simulink model "s2_0515"  (R2016a)
settings: Solver=ode23tb  StartTime=0.0  StopTime=40e-6  MaxStep=0.2  RelTol=1e-4
PreLoadFcn:
  | % -- Recommended Settings --
  | %
  | %  Simulink:
  | %      Solver: Ode23tb
  | %      Relative tolerance = 1e-4
  | %      Max step size = 0.2
  | %
  | %  Powergui:
  |          Ts = 0; % (continuous electrical model)
  | %
  | %
  | % ----------------------------------
libraries: powerlib x14
settings Model: Creator=Administrator  LastModifiedBy=Administrator
settings DataIOCC: LimitDataPoints=on
settings DebuggingCC: AllowSymbolicDim=off
settings ConfigComp: CovModelRefEnable=Off  CovSFcnEnable=off

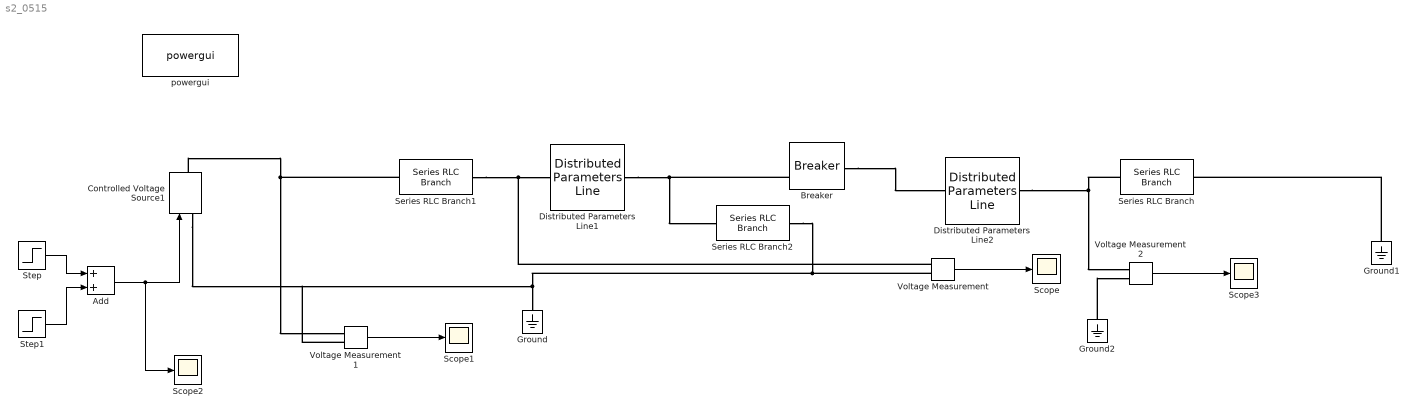
== system s2_0515 ==
  Add : Sum
  Breaker : powerlib/Elements/Breaker  InitialState=1  SwitchingTimes="[1/60  5/60]"  External=on  BreakerResistance=0.01  SnubberResistance=1e6  SnubberCapacitance=inf  Measurements=None  MoreParameters=on  NoBreakLoop=off
  Controlled Voltage Source1 : powerlib/Electrical Sources/Controlled Voltage Source  Initialize=off  Source_Type=DC  Amplitude=0  Phase=0  Frequency=0  Measurements=Voltage
  Distributed Parameters Line1 : powerlib/Elements/Distributed Parameters Line  Phases=1  Frequency=1000  Resistance=1.8E-1  Inductance=2.75E-4  Capacitance=5.57E-7  Length=0.2  x1=[-2.48e-06 0;-2.47e-06 0;-2.46e-06 0;-2.45e-06 0;-2.44e-06 0;-2.43e-06 0;-2.42e-06 0;-2.41e-06 0;-2.4e-06 0;-2.39e-06 0;-2.38e-06 0;-2.37e-06 0;-2.36e-06 0;-2.35e-06 0;-2.34e-06 0;-2.33e-06 0;-2.32e-06 0;-2.31e-06 0;-2.3e-06 0;-2.29e-06 0;-2.28e-06 0;-2.27e-06 0;-2.26e-06 0;-2.25e-06 0;-2.24e-06 0;-2.23e-06 0;-2.22e-06 0;-2.21e-06 0;-2.2e-06 0;-2.19e-06 0;-2.18e-06 0;-2.17e-06 0;-2.16e-06 0;-2.15e-06 0;-2.14e-06 0;-2.13e-06 0;-2.12e-06 0;-2.11e-06 0;-2.1e-06 0;-2.09e-06 0;-2.08e-06 0;-2.07e-06 0;-2.06e-06 0;-2.05e-06 0;-2.04e-06 0;-2.03e-06 0;-2.02e-06 0;-2.01e-06 0;-2e-06 0;-1.99e-06 0;-1.98e-06 0;-1.97e-06 0;-1.96e-06 0;-1.95e-06 0;-1.94e-06 0;-1.93e-06 0;-1.92e-06 0;-1.91e-06 0;-1.9e-06 0;-1.89e-06 0;-1.88e-06 0;-1.87e-06 0;-1.86e-06 0;-1.85e-06 0;-1.84e-06 0;-1.83e-06 0;-1.82e-06 0;-1.81e-06 0;-1.8e-06 0;-1.79e-06 0;-1.78e-06 0;-1.77e-06 0;-1.76e-06 0;-1.75e-06 0;-1.74e-06 0;-1.73e-06 0;-1.72e-06 0;-1.71e-06 0;-1.7e-06 0;-1.69e-06 0;-1.68e-06 0;-1.67e-06 0;-1.66e-06 0;-1.65e-06 0;-1.64e-06 0;-1.63e-06 0;-1.62e-06 0;-1.61e-06 0;-1.6e-06 0;-1.59e-06 0;-1.58e-06 0;-1.57e-06 0;-1.56e-06 0;-1.55e-06 0;-1.54e-06 0;-1.53e-06 0;-1.52e-06 0;-1.51e-06 0;-1.5e-06 0;-1.49e-06 0;-1.48e-06 0;-1.47e-06 0;-1.46e-06 0;-1.45e-06 0;-1.44e-06 0;-1.43e-06 0;-1.42e-06 0;-1.41e-06 0;-1.4e-06 0;-1.39e-06 0;-1.38e-06 0;-1.37e-06 0;-1.36e-06 0;-1.35e-06 0;-1.34e-06 0;-1.33e-06 0;-1.32e-06 0;-1.31e-06 0;-1.3e-06 0;-1.29e-06 0;-1.28e-06 0;-1.27e-06 0;-1.26e-06 0;-1.25e-06 0;-1.24e-06 0;-1.23e-06 0;-1.22e-06 0;-1.21e-06 0;-1.2e-06 0;-1.19e-06 0;-1.18e-06 0;-1.17e-06 0;-1.16e-06 0;-1.15e-06 0;-1.14e-06 0;-1.13e-06 0;-1.12e-06 0;-1.11e-06 0;-1.1e-06 0;-1.09e-06 0;-1.08e-06 0;-1.07e-06 0;-1.06e-06 0;-1.05e-06 0;-1.04e-06 0;-1.03e-06 0;-1.02e-06 0;-1.01e-06 0;-1e-06 0;-9.9e-07 0;-9.8e-07 0;-9.7e-07 0;-9.6e-07 0;-9.5e-07 0;-9.4e-07 0;-9.3e-07 0;-9.2e-07 0;-9.1e-07 0;-9e-07 0;-8.9e-07 0;-8.8e-07 0;-8.7e-07 0;-8.6e-07 0;-8.5e-07 0;-8.4e-07 0;-8.3e-07 0;-8.2e-07 0;-8.1e-07 0;-8e-07 0;-7.9e-07 0;-7.8e-07 0;-7.7e-07 0;-7.6e-07 0;-7.5e-07 0;-7.4e-07 0;-7.3e-07 0;-7.2e-07 0;-7.1e-07 0;-7e-07 0;-6.9e-07 0;-6.8e-07 0;-6.7e-07 0;-6.6e-07 0;-6.5e-07 0;-6.4e-07 0;-6.3e-07 0;-6.2e-07 0;-6.1e-07 0;-6e-07 0;-5.9e-07 0;-5.8e-07 0;-5.7e-07 0;-5.6e-07 0;-5.5e-07 0;-5.4e-07 0;-5.3e-07 0;-5.2e-07 0;-5.1e-07 0;-5e-07 0;-4.9e-07 0;-4.8e-07 0;-4.7e-07 0;-4.6e-07 0;-4.5e-07 0;-4.4e-07 0;-4.3e-07 0;-4.2e-07 0;-4.1e-07 0;-4e-07 0;-3.9e-07 0;-3.8e-07 0;-3.7e-07 0;-3.6e-07 0;-3.5e-07 0;-3.4e-07 0;-3.3e-07 0;-3.2e-07 0;-3.1e-07 0;-3e-07 0;-2.9e-07 0;-2.8e-07 0;-2.7e-07 0;-2.6e-07 0;-2.5e-07 0;-2.4e-07 0;-2.3e-07 0;-2.2e-07 0;-2.1e-07 0;-2e-07 0;-1.9e-07 0;-1.8e-07 0;-1.7e-07 0;-1.6e-07 0;-1.5e-07 0;-1.4e-07 0;-1.3e-07 0;-1.2e-07 0;-1.1e-07 0;-1e-07 0;-9e-08 0;-8e-08 0;-7e-08 0;-6e-08 0;-5e-08 0;-4e-08 0;-3e-08 0;-2e-08 0;-1e-08 0]  x2=[-2.48e-06 0;-2.47e-06 0;-2.46e-06 0;-2.45e-06 0;-2.44e-06 0;-2.43e-06 0;-2.42e-06 0;-2.41e-06 0;-2.4e-06 0;-2.39e-06 0;-2.38e-06 0;-2.37e-06 0;-2.36e-06 0;-2.35e-06 0;-2.34e-06 0;-2.33e-06 0;-2.32e-06 0;-2.31e-06 0;-2.3e-06 0;-2.29e-06 0;-2.28e-06 0;-2.27e-06 0;-2.26e-06 0;-2.25e-06 0;-2.24e-06 0;-2.23e-06 0;-2.22e-06 0;-2.21e-06 0;-2.2e-06 0;-2.19e-06 0;-2.18e-06 0;-2.17e-06 0;-2.16e-06 0;-2.15e-06 0;-2.14e-06 0;-2.13e-06 0;-2.12e-06 0;-2.11e-06 0;-2.1e-06 0;-2.09e-06 0;-2.08e-06 0;-2.07e-06 0;-2.06e-06 0;-2.05e-06 0;-2.04e-06 0;-2.03e-06 0;-2.02e-06 0;-2.01e-06 0;-2e-06 0;-1.99e-06 0;-1.98e-06 0;-1.97e-06 0;-1.96e-06 0;-1.95e-06 0;-1.94e-06 0;-1.93e-06 0;-1.92e-06 0;-1.91e-06 0;-1.9e-06 0;-1.89e-06 0;-1.88e-06 0;-1.87e-06 0;-1.86e-06 0;-1.85e-06 0;-1.84e-06 0;-1.83e-06 0;-1.82e-06 0;-1.81e-06 0;-1.8e-06 0;-1.79e-06 0;-1.78e-06 0;-1.77e-06 0;-1.76e-06 0;-1.75e-06 0;-1.74e-06 0;-1.73e-06 0;-1.72e-06 0;-1.71e-06 0;-1.7e-06 0;-1.69e-06 0;-1.68e-06 0;-1.67e-06 0;-1.66e-06 0;-1.65e-06 0;-1.64e-06 0;-1.63e-06 0;-1.62e-06 0;-1.61e-06 0;-1.6e-06 0;-1.59e-06 0;-1.58e-06 0;-1.57e-06 0;-1.56e-06 0;-1.55e-06 0;-1.54e-06 0;-1.53e-06 0;-1.52e-06 0;-1.51e-06 0;-1.5e-06 0;-1.49e-06 0;-1.48e-06 0;-1.47e-06 0;-1.46e-06 0;-1.45e-06 0;-1.44e-06 0;-1.43e-06 0;-1.42e-06 0;-1.41e-06 0;-1.4e-06 0;-1.39e-06 0;-1.38e-06 0;-1.37e-06 0;-1.36e-06 0;-1.35e-06 0;-1.34e-06 0;-1.33e-06 0;-1.32e-06 0;-1.31e-06 0;-1.3e-06 0;-1.29e-06 0;-1.28e-06 0;-1.27e-06 0;-1.26e-06 0;-1.25e-06 0;-1.24e-06 0;-1.23e-06 0;-1.22e-06 0;-1.21e-06 0;-1.2e-06 0;-1.19e-06 0;-1.18e-06 0;-1.17e-06 0;-1.16e-06 0;-1.15e-06 0;-1.14e-06 0;-1.13e-06 0;-1.12e-06 0;-1.11e-06 0;-1.1e-06 0;-1.09e-06 0;-1.08e-06 0;-1.07e-06 0;-1.06e-06 0;-1.05e-06 0;-1.04e-06 0;-1.03e-06 0;-1.02e-06 0;-1.01e-06 0;-1e-06 0;-9.9e-07 0;-9.8e-07 0;-9.7e-07 0;-9.6e-07 0;-9.5e-07 0;-9.4e-07 0;-9.3e-07 0;-9.2e-07 0;-9.1e-07 0;-9e-07 0;-8.9e-07 0;-8.8e-07 0;-8.7e-07 0;-8.6e-07 0;-8.5e-07 0;-8.4e-07 0;-8.3e-07 0;-8.2e-07 0;-8.1e-07 0;-8e-07 0;-7.9e-07 0;-7.8e-07 0;-7.7e-07 0;-7.6e-07 0;-7.5e-07 0;-7.4e-07 0;-7.3e-07 0;-7.2e-07 0;-7.1e-07 0;-7e-07 0;-6.9e-07 0;-6.8e-07 0;-6.7e-07 0;-6.6e-07 0;-6.5e-07 0;-6.4e-07 0;-6.3e-07 0;-6.2e-07 0;-6.1e-07 0;-6e-07 0;-5.9e-07 0;-5.8e-07 0;-5.7e-07 0;-5.6e-07 0;-5.5e-07 0;-5.4e-07 0;-5.3e-07 0;-5.2e-07 0;-5.1e-07 0;-5e-07 0;-4.9e-07 0;-4.8e-07 0;-4.7e-07 0;-4.6e-07 0;-4.5e-07 0;-4.4e-07 0;-4.3e-07 0;-4.2e-07 0;-4.1e-07 0;-4e-07 0;-3.9e-07 0;-3.8e-07 0;-3.7e-07 0;-3.6e-07 0;-3.5e-07 0;-3.4e-07 0;-3.3e-07 0;-3.2e-07 0;-3.1e-07 0;-3e-07 0;-2.9e-07 0;-2.8e-07 0;-2.7e-07 0;-2.6e-07 0;-2.5e-07 0;-2.4e-07 0;-2.3e-07 0;-2.2e-07 0;-2.1e-07 0;-2e-07 0;-1.9e-07 0;-1.8e-07 0;-1.7e-07 0;-1.6e-07 0;-1.5e-07 0;-1.4e-07 0;-1.3e-07 0;-1.2e-07 0;-1.1e-07 0;-1e-07 0;-9e-08 0;-8e-08 0;-7e-08 0;-6e-08 0;-5e-08 0;-4e-08 0;-3e-08 0;-2e-08 0;-1e-08 0]  x3=[-2.48e-06 0;-2.47e-06 0;-2.46e-06 0;-2.45e-06 0;-2.44e-06 0;-2.43e-06 0;-2.42e-06 0;-2.41e-06 0;-2.4e-06 0;-2.39e-06 0;-2.38e-06 0;-2.37e-06 0;-2.36e-06 0;-2.35e-06 0;-2.34e-06 0;-2.33e-06 0;-2.32e-06 0;-2.31e-06 0;-2.3e-06 0;-2.29e-06 0;-2.28e-06 0;-2.27e-06 0;-2.26e-06 0;-2.25e-06 0;-2.24e-06 0;-2.23e-06 0;-2.22e-06 0;-2.21e-06 0;-2.2e-06 0;-2.19e-06 0;-2.18e-06 0;-2.17e-06 0;-2.16e-06 0;-2.15e-06 0;-2.14e-06 0;-2.13e-06 0;-2.12e-06 0;-2.11e-06 0;-2.1e-06 0;-2.09e-06 0;-2.08e-06 0;-2.07e-06 0;-2.06e-06 0;-2.05e-06 0;-2.04e-06 0;-2.03e-06 0;-2.02e-06 0;-2.01e-06 0;-2e-06 0;-1.99e-06 0;-1.98e-06 0;-1.97e-06 0;-1.96e-06 0;-1.95e-06 0;-1.94e-06 0;-1.93e-06 0;-1.92e-06 0;-1.91e-06 0;-1.9e-06 0;-1.89e-06 0;-1.88e-06 0;-1.87e-06 0;-1.86e-06 0;-1.85e-06 0;-1.84e-06 0;-1.83e-06 0;-1.82e-06 0;-1.81e-06 0;-1.8e-06 0;-1.79e-06 0;-1.78e-06 0;-1.77e-06 0;-1.76e-06 0;-1.75e-06 0;-1.74e-06 0;-1.73e-06 0;-1.72e-06 0;-1.71e-06 0;-1.7e-06 0;-1.69e-06 0;-1.68e-06 0;-1.67e-06 0;-1.66e-06 0;-1.65e-06 0;-1.64e-06 0;-1.63e-06 0;-1.62e-06 0;-1.61e-06 0;-1.6e-06 0;-1.59e-06 0;-1.58e-06 0;-1.57e-06 0;-1.56e-06 0;-1.55e-06 0;-1.54e-06 0;-1.53e-06 0;-1.52e-06 0;-1.51e-06 0;-1.5e-06 0;-1.49e-06 0;-1.48e-06 0;-1.47e-06 0;-1.46e-06 0;-1.45e-06 0;-1.44e-06 0;-1.43e-06 0;-1.42e-06 0;-1.41e-06 0;-1.4e-06 0;-1.39e-06 0;-1.38e-06 0;-1.37e-06 0;-1.36e-06 0;-1.35e-06 0;-1.34e-06 0;-1.33e-06 0;-1.32e-06 0;-1.31e-06 0;-1.3e-06 0;-1.29e-06 0;-1.28e-06 0;-1.27e-06 0;-1.26e-06 0;-1.25e-06 0;-1.24e-06 0;-1.23e-06 0;-1.22e-06 0;-1.21e-06 0;-1.2e-06 0;-1.19e-06 0;-1.18e-06 0;-1.17e-06 0;-1.16e-06 0;-1.15e-06 0;-1.14e-06 0;-1.13e-06 0;-1.12e-06 0;-1.11e-06 0;-1.1e-06 0;-1.09e-06 0;-1.08e-06 0;-1.07e-06 0;-1.06e-06 0;-1.05e-06 0;-1.04e-06 0;-1.03e-06 0;-1.02e-06 0;-1.01e-06 0;-1e-06 0;-9.9e-07 0;-9.8e-07 0;-9.7e-07 0;-9.6e-07 0;-9.5e-07 0;-9.4e-07 0;-9.3e-07 0;-9.2e-07 0;-9.1e-07 0;-9e-07 0;-8.9e-07 0;-8.8e-07 0;-8.7e-07 0;-8.6e-07 0;-8.5e-07 0;-8.4e-07 0;-8.3e-07 0;-8.2e-07 0;-8.1e-07 0;-8e-07 0;-7.9e-07 0;-7.8e-07 0;-7.7e-07 0;-7.6e-07 0;-7.5e-07 0;-7.4e-07 0;-7.3e-07 0;-7.2e-07 0;-7.1e-07 0;-7e-07 0;-6.9e-07 0;-6.8e-07 0;-6.7e-07 0;-6.6e-07 0;-6.5e-07 0;-6.4e-07 0;-6.3e-07 0;-6.2e-07 0;-6.1e-07 0;-6e-07 0;-5.9e-07 0;-5.8e-07 0;-5.7e-07 0;-5.6e-07 0;-5.5e-07 0;-5.4e-07 0;-5.3e-07 0;-5.2e-07 0;-5.1e-07 0;-5e-07 0;-4.9e-07 0;-4.8e-07 0;-4.7e-07 0;-4.6e-07 0;-4.5e-07 0;-4.4e-07 0;-4.3e-07 0;-4.2e-07 0;-4.1e-07 0;-4e-07 0;-3.9e-07 0;-3.8e-07 0;-3.7e-07 0;-3.6e-07 0;-3.5e-07 0;-3.4e-07 0;-3.3e-07 0;-3.2e-07 0;-3.1e-07 0;-3e-07 0;-2.9e-07 0;-2.8e-07 0;-2.7e-07 0;-2.6e-07 0;-2.5e-07 0;-2.4e-07 0;-2.3e-07 0;-2.2e-07 0;-2.1e-07 0;-2e-07 0;-1.9e-07 0;-1.8e-07 0;-1.7e-07 0;-1.6e-07 0;-1.5e-07 0;-1.4e-07 0;-1.3e-07 0;-1.2e-07 0;-1.1e-07 0;-1e-07 0;-9e-08 0;-8e-08 0;-7e-08 0;-6e-08 0;-5e-08 0;-4e-08 0;-3e-08 0;-2e-08 0;-1e-08 0]  x4=[-2.48e-06 0;-2.47e-06 0;-2.46e-06 0;-2.45e-06 0;-2.44e-06 0;-2.43e-06 0;-2.42e-06 0;-2.41e-06 0;-2.4e-06 0;-2.39e-06 0;-2.38e-06 0;-2.37e-06 0;-2.36e-06 0;-2.35e-06 0;-2.34e-06 0;-2.33e-06 0;-2.32e-06 0;-2.31e-06 0;-2.3e-06 0;-2.29e-06 0;-2.28e-06 0;-2.27e-06 0;-2.26e-06 0;-2.25e-06 0;-2.24e-06 0;-2.23e-06 0;-2.22e-06 0;-2.21e-06 0;-2.2e-06 0;-2.19e-06 0;-2.18e-06 0;-2.17e-06 0;-2.16e-06 0;-2.15e-06 0;-2.14e-06 0;-2.13e-06 0;-2.12e-06 0;-2.11e-06 0;-2.1e-06 0;-2.09e-06 0;-2.08e-06 0;-2.07e-06 0;-2.06e-06 0;-2.05e-06 0;-2.04e-06 0;-2.03e-06 0;-2.02e-06 0;-2.01e-06 0;-2e-06 0;-1.99e-06 0;-1.98e-06 0;-1.97e-06 0;-1.96e-06 0;-1.95e-06 0;-1.94e-06 0;-1.93e-06 0;-1.92e-06 0;-1.91e-06 0;-1.9e-06 0;-1.89e-06 0;-1.88e-06 0;-1.87e-06 0;-1.86e-06 0;-1.85e-06 0;-1.84e-06 0;-1.83e-06 0;-1.82e-06 0;-1.81e-06 0;-1.8e-06 0;-1.79e-06 0;-1.78e-06 0;-1.77e-06 0;-1.76e-06 0;-1.75e-06 0;-1.74e-06 0;-1.73e-06 0;-1.72e-06 0;-1.71e-06 0;-1.7e-06 0;-1.69e-06 0;-1.68e-06 0;-1.67e-06 0;-1.66e-06 0;-1.65e-06 0;-1.64e-06 0;-1.63e-06 0;-1.62e-06 0;-1.61e-06 0;-1.6e-06 0;-1.59e-06 0;-1.58e-06 0;-1.57e-06 0;-1.56e-06 0;-1.55e-06 0;-1.54e-06 0;-1.53e-06 0;-1.52e-06 0;-1.51e-06 0;-1.5e-06 0;-1.49e-06 0;-1.48e-06 0;-1.47e-06 0;-1.46e-06 0;-1.45e-06 0;-1.44e-06 0;-1.43e-06 0;-1.42e-06 0;-1.41e-06 0;-1.4e-06 0;-1.39e-06 0;-1.38e-06 0;-1.37e-06 0;-1.36e-06 0;-1.35e-06 0;-1.34e-06 0;-1.33e-06 0;-1.32e-06 0;-1.31e-06 0;-1.3e-06 0;-1.29e-06 0;-1.28e-06 0;-1.27e-06 0;-1.26e-06 0;-1.25e-06 0;-1.24e-06 0;-1.23e-06 0;-1.22e-06 0;-1.21e-06 0;-1.2e-06 0;-1.19e-06 0;-1.18e-06 0;-1.17e-06 0;-1.16e-06 0;-1.15e-06 0;-1.14e-06 0;-1.13e-06 0;-1.12e-06 0;-1.11e-06 0;-1.1e-06 0;-1.09e-06 0;-1.08e-06 0;-1.07e-06 0;-1.06e-06 0;-1.05e-06 0;-1.04e-06 0;-1.03e-06 0;-1.02e-06 0;-1.01e-06 0;-1e-06 0;-9.9e-07 0;-9.8e-07 0;-9.7e-07 0;-9.6e-07 0;-9.5e-07 0;-9.4e-07 0;-9.3e-07 0;-9.2e-07 0;-9.1e-07 0;-9e-07 0;-8.9e-07 0;-8.8e-07 0;-8.7e-07 0;-8.6e-07 0;-8.5e-07 0;-8.4e-07 0;-8.3e-07 0;-8.2e-07 0;-8.1e-07 0;-8e-07 0;-7.9e-07 0;-7.8e-07 0;-7.7e-07 0;-7.6e-07 0;-7.5e-07 0;-7.4e-07 0;-7.3e-07 0;-7.2e-07 0;-7.1e-07 0;-7e-07 0;-6.9e-07 0;-6.8e-07 0;-6.7e-07 0;-6.6e-07 0;-6.5e-07 0;-6.4e-07 0;-6.3e-07 0;-6.2e-07 0;-6.1e-07 0;-6e-07 0;-5.9e-07 0;-5.8e-07 0;-5.7e-07 0;-5.6e-07 0;-5.5e-07 0;-5.4e-07 0;-5.3e-07 0;-5.2e-07 0;-5.1e-07 0;-5e-07 0;-4.9e-07 0;-4.8e-07 0;-4.7e-07 0;-4.6e-07 0;-4.5e-07 0;-4.4e-07 0;-4.3e-07 0;-4.2e-07 0;-4.1e-07 0;-4e-07 0;-3.9e-07 0;-3.8e-07 0;-3.7e-07 0;-3.6e-07 0;-3.5e-07 0;-3.4e-07 0;-3.3e-07 0;-3.2e-07 0;-3.1e-07 0;-3e-07 0;-2.9e-07 0;-2.8e-07 0;-2.7e-07 0;-2.6e-07 0;-2.5e-07 0;-2.4e-07 0;-2.3e-07 0;-2.2e-07 0;-2.1e-07 0;-2e-07 0;-1.9e-07 0;-1.8e-07 0;-1.7e-07 0;-1.6e-07 0;-1.5e-07 0;-1.4e-07 0;-1.3e-07 0;-1.2e-07 0;-1.1e-07 0;-1e-07 0;-9e-08 0;-8e-08 0;-7e-08 0;-6e-08 0;-5e-08 0;-4e-08 0;-3e-08 0;-2e-08 0;-1e-08 0]  x5=2.47527776219155e-06  V1=[0;0;1.571]  V2=[0;0;1.571]  I1=[0;0;1.571]  I2=[0;0;1.571]  nHarmo=1  Measurements=Phase-to-ground voltages
  Distributed Parameters Line2 : powerlib/Elements/Distributed Parameters Line  Phases=1  Frequency=1000  Resistance=1.8E-1  Inductance=2.75E-4  Capacitance=5.57E-7  Length=0.8  x1=[-9.91e-06 0;-9.9e-06 0;-9.89e-06 0;-9.88e-06 0;-9.87e-06 0;-9.86e-06 0;-9.85e-06 0;-9.84e-06 0;-9.83e-06 0;-9.82e-06 0;-9.81e-06 0;-9.8e-06 0;-9.79e-06 0;-9.78e-06 0;-9.77e-06 0;-9.76e-06 0;-9.75e-06 0;-9.74e-06 0;-9.73e-06 0;-9.72e-06 0;-9.71e-06 0;-9.7e-06 0;-9.69e-06 0;-9.68e-06 0;-9.67e-06 0;-9.66e-06 0;-9.65e-06 0;-9.64e-06 0;-9.63e-06 0;-9.62e-06 0;-9.61e-06 0;-9.6e-06 0;-9.59e-06 0;-9.58e-06 0;-9.57e-06 0;-9.56e-06 0;-9.55e-06 0;-9.54e-06 0;-9.53e-06 0;-9.52e-06 0;-9.51e-06 0;-9.5e-06 0;-9.49e-06 0;-9.48e-06 0;-9.47e-06 0;-9.46e-06 0;-9.45e-06 0;-9.44e-06 0;-9.43e-06 0;-9.42e-06 0;-9.41e-06 0;-9.4e-06 0;-9.39e-06 0;-9.38e-06 0;-9.37e-06 0;-9.36e-06 0;-9.35e-06 0;-9.34e-06 0;-9.33e-06 0;-9.32e-06 0;-9.31e-06 0;-9.3e-06 0;-9.29e-06 0;-9.28e-06 0;-9.27e-06 0;-9.26e-06 0;-9.25e-06 0;-9.24e-06 0;-9.23e-06 0;-9.22e-06 0;-9.21e-06 0;-9.2e-06 0;-9.19e-06 0;-9.18e-06 0;-9.17e-06 0;-9.16e-06 0;-9.15e-06 0;-9.14e-06 0;-9.13e-06 0;-9.12e-06 0;-9.11e-06 0;-9.1e-06 0;-9.09e-06 0;-9.08e-06 0;-9.07e-06 0;-9.06e-06 0;-9.05e-06 0;-9.04e-06 0;-9.03e-06 0;-9.02e-06 0;-9.01e-06 0;-9e-06 0;-8.99e-06 0;-8.98e-06 0;-8.97e-06 0;-8.96e-06 0;-8.95e-06 0;-8.94e-06 0;-8.93e-06 0;-8.92e-06 0;-8.91e-06 0;-8.9e-06 0;-8.89e-06 0;-8.88e-06 0;-8.87e-06 0;-8.86e-06 0;-8.85e-06 0;-8.84e-06 0;-8.83e-06 0;-8.82e-06 0;-8.81e-06 0;-8.8e-06 0;-8.79e-06 0;-8.78e-06 0;-8.77e-06 0;-8.76e-06 0;-8.75e-06 0;-8.74e-06 0;-8.73e-06 0;-8.72e-06 0;-8.71e-06 0;-8.7e-06 0;-8.69e-06 0;-8.68e-06 0;-8.67e-06 0;-8.66e-06 0;-8.65e-06 0;-8.64e-06 0;-8.63e-06 0;-8.62e-06 0;-8.61e-06 0;-8.6e-06 0;-8.59e-06 0;-8.58e-06 0;-8.57e-06 0;-8.56e-06 0;-8.55e-06 0;-8.54e-06 0;-8.53e-06 0;-8.52e-06 0;-8.51e-06 0;-8.5e-06 0;-8.49e-06 0;-8.48e-06 0;-8.47e-06 0;-8.46e-06 0;-8.45e-06 0;-8.44e-06 0;-8.43e-06 0;-8.42e-06 0;-8.41e-06 0;-8.4e-06 0;-8.39e-06 0;-8.38e-06 0;-8.37e-06 0;-8.36e-06 0;-8.35e-06 0;-8.34e-06 0;-8.33e-06 0;-8.32e-06 0;-8.31e-06 0;-8.3e-06 0;-8.29e-06 0;-8.28e-06 0;-8.27e-06 0;-8.26e-06 0;-8.25e-06 0;-8.24e-06 0;-8.23e-06 0;-8.22e-06 0;-8.21e-06 0;-8.2e-06 0;-8.19e-06 0;-8.18e-06 0;-8.17e-06 0;-8.16e-06 0;-8.15e-06 0;-8.14e-06 0;-8.13e-06 0;-8.12e-06 0;-8.11e-06 0;-8.1e-06 0;-8.09e-06 0;-8.08e-06 0;-8.07e-06 0;-8.06e-06 0;-8.05e-06 0;-8.04e-06 0;-8.03e-06 0;-8.02e-06 0;-8.01e-06 0;-8e-06 0;-7.99e-06 0;-7.98e-06 0;-7.97e-06 0;-7.96e-06 0;-7.95e-06 0;-7.94e-06 0;-7.93e-06 0;-7.92e-06 0;-7.91e-06 0;-7.9e-06 0;-7.89e-06 0;-7.88e-06 0;-7.87e-06 0;-7.86e-06 0;-7.85e-06 0;-7.84e-06 0;-7.83e-06 0;-7.82e-06 0;-7.81e-06 0;-7.8e-06 0;-7.79e-06 0;-7.78e-06 0;-7.77e-06 0;-7.76e-06 0;-7.75e-06 0;-7.74e-06 0;-7.73e-06 0;-7.72e-06 0;-7.71e-06 0;-7.7e-06 0;-7.69e-06 0;-7.68e-06 0;-7.67e-06 0;-7.66e-06 0;-7.65e-06 0;-7.64e-06 0;-7.63e-06 0;-7.62e-06 0;-7.61e-06 0;-7.6e-06 0;-7.59e-06 0;-7.58e-06 0;-7.57e-06 0;-7.56e-06 0;-7.55e-06 0;-7.54e-06 0;-7.53e-06 0;-7.52e-06 0;-7.51e-06 0;-7.5e-06 0;-7.49e-06 0;-7.48e-06 0;-7.47e-06 0;-7.46e-06 0;-7.45e-06 0;-7.44e-06 0;-7.43e-06 0;-7.42e-06 0;-7.41e-06 0;-7.4e-06 0;-7.39e-06 0;-7.38e-06 0;-7.37e-06 0;-7.36e-06 0;-7.35e-06 0;-7.34e-06 0;-7.33e-06 0;-7.32e-06 0;-7.31e-06 0;-7.3e-06 0;-7.29e-06 0;-7.28e-06 0;-7.27e-06 0;-7.26e-06 0;-7.25e-06 0;-7.24e-06 0;-7.23e-06 0;-7.22e-06 0;-7.21e-06 0;-7.2e-06 0;-7.19e-06 0;-7.18e-06 0;-7.17e-06 0;-7.16e-06 0;-7.15e-06 0;-7.14e-06 0;-7.13e-06 0;-7.12e-06 0;-7.11e-06 0;-7.1e-06 0;-7.09e-06 0;-7.08e-06 0;-7.07e-06 0;-7.06e-06 0;-7.05e-06 0;-7.04e-06 0;-7.03e-06 0;-7.02e-06 0;-7.01e-06 0;-7e-06 0;-6.99e-06 0;-6.98e-06 0;-6.97e-06 0;-6.96e-06 0;-6.95e-06 0;-6.94e-06 0;-6.93e-06 0;-6.92e-06 0;-6.91e-06 0;-6.9e-06 0;-6.89e-06 0;-6.88e-06 0;-6.87e-06 0;-6.86e-06 0;-6.85e-06 0;-6.84e-06 0;-6.83e-06 0;-6.82e-06 0;-6.81e-06 0;-6.8e-06 0;-6.79e-06 0;-6.78e-06 0;-6.77e-06 0;-6.76e-06 0;-6.75e-06 0;-6.74e-06 0;-6.73e-06 0;-6.72e-06 0;-6.71e-06 0;-6.7e-06 0;-6.69e-06 0;-6.68e-06 0;-6.67e-06 0;-6.66e-06 0;-6.65e-06 0;-6.64e-06 0;-6.63e-06 0;-6.62e-06 0;-6.61e-06 0;-6.6e-06 0;-6.59e-06 0;-6.58e-06 0;-6.57e-06 0;-6.56e-06 0 ...(+7657 chars)]  x2=[-9.91e-06 0;-9.9e-06 0;-9.89e-06 0;-9.88e-06 0;-9.87e-06 0;-9.86e-06 0;-9.85e-06 0;-9.84e-06 0;-9.83e-06 0;-9.82e-06 0;-9.81e-06 0;-9.8e-06 0;-9.79e-06 0;-9.78e-06 0;-9.77e-06 0;-9.76e-06 0;-9.75e-06 0;-9.74e-06 0;-9.73e-06 0;-9.72e-06 0;-9.71e-06 0;-9.7e-06 0;-9.69e-06 0;-9.68e-06 0;-9.67e-06 0;-9.66e-06 0;-9.65e-06 0;-9.64e-06 0;-9.63e-06 0;-9.62e-06 0;-9.61e-06 0;-9.6e-06 0;-9.59e-06 0;-9.58e-06 0;-9.57e-06 0;-9.56e-06 0;-9.55e-06 0;-9.54e-06 0;-9.53e-06 0;-9.52e-06 0;-9.51e-06 0;-9.5e-06 0;-9.49e-06 0;-9.48e-06 0;-9.47e-06 0;-9.46e-06 0;-9.45e-06 0;-9.44e-06 0;-9.43e-06 0;-9.42e-06 0;-9.41e-06 0;-9.4e-06 0;-9.39e-06 0;-9.38e-06 0;-9.37e-06 0;-9.36e-06 0;-9.35e-06 0;-9.34e-06 0;-9.33e-06 0;-9.32e-06 0;-9.31e-06 0;-9.3e-06 0;-9.29e-06 0;-9.28e-06 0;-9.27e-06 0;-9.26e-06 0;-9.25e-06 0;-9.24e-06 0;-9.23e-06 0;-9.22e-06 0;-9.21e-06 0;-9.2e-06 0;-9.19e-06 0;-9.18e-06 0;-9.17e-06 0;-9.16e-06 0;-9.15e-06 0;-9.14e-06 0;-9.13e-06 0;-9.12e-06 0;-9.11e-06 0;-9.1e-06 0;-9.09e-06 0;-9.08e-06 0;-9.07e-06 0;-9.06e-06 0;-9.05e-06 0;-9.04e-06 0;-9.03e-06 0;-9.02e-06 0;-9.01e-06 0;-9e-06 0;-8.99e-06 0;-8.98e-06 0;-8.97e-06 0;-8.96e-06 0;-8.95e-06 0;-8.94e-06 0;-8.93e-06 0;-8.92e-06 0;-8.91e-06 0;-8.9e-06 0;-8.89e-06 0;-8.88e-06 0;-8.87e-06 0;-8.86e-06 0;-8.85e-06 0;-8.84e-06 0;-8.83e-06 0;-8.82e-06 0;-8.81e-06 0;-8.8e-06 0;-8.79e-06 0;-8.78e-06 0;-8.77e-06 0;-8.76e-06 0;-8.75e-06 0;-8.74e-06 0;-8.73e-06 0;-8.72e-06 0;-8.71e-06 0;-8.7e-06 0;-8.69e-06 0;-8.68e-06 0;-8.67e-06 0;-8.66e-06 0;-8.65e-06 0;-8.64e-06 0;-8.63e-06 0;-8.62e-06 0;-8.61e-06 0;-8.6e-06 0;-8.59e-06 0;-8.58e-06 0;-8.57e-06 0;-8.56e-06 0;-8.55e-06 0;-8.54e-06 0;-8.53e-06 0;-8.52e-06 0;-8.51e-06 0;-8.5e-06 0;-8.49e-06 0;-8.48e-06 0;-8.47e-06 0;-8.46e-06 0;-8.45e-06 0;-8.44e-06 0;-8.43e-06 0;-8.42e-06 0;-8.41e-06 0;-8.4e-06 0;-8.39e-06 0;-8.38e-06 0;-8.37e-06 0;-8.36e-06 0;-8.35e-06 0;-8.34e-06 0;-8.33e-06 0;-8.32e-06 0;-8.31e-06 0;-8.3e-06 0;-8.29e-06 0;-8.28e-06 0;-8.27e-06 0;-8.26e-06 0;-8.25e-06 0;-8.24e-06 0;-8.23e-06 0;-8.22e-06 0;-8.21e-06 0;-8.2e-06 0;-8.19e-06 0;-8.18e-06 0;-8.17e-06 0;-8.16e-06 0;-8.15e-06 0;-8.14e-06 0;-8.13e-06 0;-8.12e-06 0;-8.11e-06 0;-8.1e-06 0;-8.09e-06 0;-8.08e-06 0;-8.07e-06 0;-8.06e-06 0;-8.05e-06 0;-8.04e-06 0;-8.03e-06 0;-8.02e-06 0;-8.01e-06 0;-8e-06 0;-7.99e-06 0;-7.98e-06 0;-7.97e-06 0;-7.96e-06 0;-7.95e-06 0;-7.94e-06 0;-7.93e-06 0;-7.92e-06 0;-7.91e-06 0;-7.9e-06 0;-7.89e-06 0;-7.88e-06 0;-7.87e-06 0;-7.86e-06 0;-7.85e-06 0;-7.84e-06 0;-7.83e-06 0;-7.82e-06 0;-7.81e-06 0;-7.8e-06 0;-7.79e-06 0;-7.78e-06 0;-7.77e-06 0;-7.76e-06 0;-7.75e-06 0;-7.74e-06 0;-7.73e-06 0;-7.72e-06 0;-7.71e-06 0;-7.7e-06 0;-7.69e-06 0;-7.68e-06 0;-7.67e-06 0;-7.66e-06 0;-7.65e-06 0;-7.64e-06 0;-7.63e-06 0;-7.62e-06 0;-7.61e-06 0;-7.6e-06 0;-7.59e-06 0;-7.58e-06 0;-7.57e-06 0;-7.56e-06 0;-7.55e-06 0;-7.54e-06 0;-7.53e-06 0;-7.52e-06 0;-7.51e-06 0;-7.5e-06 0;-7.49e-06 0;-7.48e-06 0;-7.47e-06 0;-7.46e-06 0;-7.45e-06 0;-7.44e-06 0;-7.43e-06 0;-7.42e-06 0;-7.41e-06 0;-7.4e-06 0;-7.39e-06 0;-7.38e-06 0;-7.37e-06 0;-7.36e-06 0;-7.35e-06 0;-7.34e-06 0;-7.33e-06 0;-7.32e-06 0;-7.31e-06 0;-7.3e-06 0;-7.29e-06 0;-7.28e-06 0;-7.27e-06 0;-7.26e-06 0;-7.25e-06 0;-7.24e-06 0;-7.23e-06 0;-7.22e-06 0;-7.21e-06 0;-7.2e-06 0;-7.19e-06 0;-7.18e-06 0;-7.17e-06 0;-7.16e-06 0;-7.15e-06 0;-7.14e-06 0;-7.13e-06 0;-7.12e-06 0;-7.11e-06 0;-7.1e-06 0;-7.09e-06 0;-7.08e-06 0;-7.07e-06 0;-7.06e-06 0;-7.05e-06 0;-7.04e-06 0;-7.03e-06 0;-7.02e-06 0;-7.01e-06 0;-7e-06 0;-6.99e-06 0;-6.98e-06 0;-6.97e-06 0;-6.96e-06 0;-6.95e-06 0;-6.94e-06 0;-6.93e-06 0;-6.92e-06 0;-6.91e-06 0;-6.9e-06 0;-6.89e-06 0;-6.88e-06 0;-6.87e-06 0;-6.86e-06 0;-6.85e-06 0;-6.84e-06 0;-6.83e-06 0;-6.82e-06 0;-6.81e-06 0;-6.8e-06 0;-6.79e-06 0;-6.78e-06 0;-6.77e-06 0;-6.76e-06 0;-6.75e-06 0;-6.74e-06 0;-6.73e-06 0;-6.72e-06 0;-6.71e-06 0;-6.7e-06 0;-6.69e-06 0;-6.68e-06 0;-6.67e-06 0;-6.66e-06 0;-6.65e-06 0;-6.64e-06 0;-6.63e-06 0;-6.62e-06 0;-6.61e-06 0;-6.6e-06 0;-6.59e-06 0;-6.58e-06 0;-6.57e-06 0;-6.56e-06 0 ...(+7657 chars)]  x3=[-9.91e-06 0;-9.9e-06 0;-9.89e-06 0;-9.88e-06 0;-9.87e-06 0;-9.86e-06 0;-9.85e-06 0;-9.84e-06 0;-9.83e-06 0;-9.82e-06 0;-9.81e-06 0;-9.8e-06 0;-9.79e-06 0;-9.78e-06 0;-9.77e-06 0;-9.76e-06 0;-9.75e-06 0;-9.74e-06 0;-9.73e-06 0;-9.72e-06 0;-9.71e-06 0;-9.7e-06 0;-9.69e-06 0;-9.68e-06 0;-9.67e-06 0;-9.66e-06 0;-9.65e-06 0;-9.64e-06 0;-9.63e-06 0;-9.62e-06 0;-9.61e-06 0;-9.6e-06 0;-9.59e-06 0;-9.58e-06 0;-9.57e-06 0;-9.56e-06 0;-9.55e-06 0;-9.54e-06 0;-9.53e-06 0;-9.52e-06 0;-9.51e-06 0;-9.5e-06 0;-9.49e-06 0;-9.48e-06 0;-9.47e-06 0;-9.46e-06 0;-9.45e-06 0;-9.44e-06 0;-9.43e-06 0;-9.42e-06 0;-9.41e-06 0;-9.4e-06 0;-9.39e-06 0;-9.38e-06 0;-9.37e-06 0;-9.36e-06 0;-9.35e-06 0;-9.34e-06 0;-9.33e-06 0;-9.32e-06 0;-9.31e-06 0;-9.3e-06 0;-9.29e-06 0;-9.28e-06 0;-9.27e-06 0;-9.26e-06 0;-9.25e-06 0;-9.24e-06 0;-9.23e-06 0;-9.22e-06 0;-9.21e-06 0;-9.2e-06 0;-9.19e-06 0;-9.18e-06 0;-9.17e-06 0;-9.16e-06 0;-9.15e-06 0;-9.14e-06 0;-9.13e-06 0;-9.12e-06 0;-9.11e-06 0;-9.1e-06 0;-9.09e-06 0;-9.08e-06 0;-9.07e-06 0;-9.06e-06 0;-9.05e-06 0;-9.04e-06 0;-9.03e-06 0;-9.02e-06 0;-9.01e-06 0;-9e-06 0;-8.99e-06 0;-8.98e-06 0;-8.97e-06 0;-8.96e-06 0;-8.95e-06 0;-8.94e-06 0;-8.93e-06 0;-8.92e-06 0;-8.91e-06 0;-8.9e-06 0;-8.89e-06 0;-8.88e-06 0;-8.87e-06 0;-8.86e-06 0;-8.85e-06 0;-8.84e-06 0;-8.83e-06 0;-8.82e-06 0;-8.81e-06 0;-8.8e-06 0;-8.79e-06 0;-8.78e-06 0;-8.77e-06 0;-8.76e-06 0;-8.75e-06 0;-8.74e-06 0;-8.73e-06 0;-8.72e-06 0;-8.71e-06 0;-8.7e-06 0;-8.69e-06 0;-8.68e-06 0;-8.67e-06 0;-8.66e-06 0;-8.65e-06 0;-8.64e-06 0;-8.63e-06 0;-8.62e-06 0;-8.61e-06 0;-8.6e-06 0;-8.59e-06 0;-8.58e-06 0;-8.57e-06 0;-8.56e-06 0;-8.55e-06 0;-8.54e-06 0;-8.53e-06 0;-8.52e-06 0;-8.51e-06 0;-8.5e-06 0;-8.49e-06 0;-8.48e-06 0;-8.47e-06 0;-8.46e-06 0;-8.45e-06 0;-8.44e-06 0;-8.43e-06 0;-8.42e-06 0;-8.41e-06 0;-8.4e-06 0;-8.39e-06 0;-8.38e-06 0;-8.37e-06 0;-8.36e-06 0;-8.35e-06 0;-8.34e-06 0;-8.33e-06 0;-8.32e-06 0;-8.31e-06 0;-8.3e-06 0;-8.29e-06 0;-8.28e-06 0;-8.27e-06 0;-8.26e-06 0;-8.25e-06 0;-8.24e-06 0;-8.23e-06 0;-8.22e-06 0;-8.21e-06 0;-8.2e-06 0;-8.19e-06 0;-8.18e-06 0;-8.17e-06 0;-8.16e-06 0;-8.15e-06 0;-8.14e-06 0;-8.13e-06 0;-8.12e-06 0;-8.11e-06 0;-8.1e-06 0;-8.09e-06 0;-8.08e-06 0;-8.07e-06 0;-8.06e-06 0;-8.05e-06 0;-8.04e-06 0;-8.03e-06 0;-8.02e-06 0;-8.01e-06 0;-8e-06 0;-7.99e-06 0;-7.98e-06 0;-7.97e-06 0;-7.96e-06 0;-7.95e-06 0;-7.94e-06 0;-7.93e-06 0;-7.92e-06 0;-7.91e-06 0;-7.9e-06 0;-7.89e-06 0;-7.88e-06 0;-7.87e-06 0;-7.86e-06 0;-7.85e-06 0;-7.84e-06 0;-7.83e-06 0;-7.82e-06 0;-7.81e-06 0;-7.8e-06 0;-7.79e-06 0;-7.78e-06 0;-7.77e-06 0;-7.76e-06 0;-7.75e-06 0;-7.74e-06 0;-7.73e-06 0;-7.72e-06 0;-7.71e-06 0;-7.7e-06 0;-7.69e-06 0;-7.68e-06 0;-7.67e-06 0;-7.66e-06 0;-7.65e-06 0;-7.64e-06 0;-7.63e-06 0;-7.62e-06 0;-7.61e-06 0;-7.6e-06 0;-7.59e-06 0;-7.58e-06 0;-7.57e-06 0;-7.56e-06 0;-7.55e-06 0;-7.54e-06 0;-7.53e-06 0;-7.52e-06 0;-7.51e-06 0;-7.5e-06 0;-7.49e-06 0;-7.48e-06 0;-7.47e-06 0;-7.46e-06 0;-7.45e-06 0;-7.44e-06 0;-7.43e-06 0;-7.42e-06 0;-7.41e-06 0;-7.4e-06 0;-7.39e-06 0;-7.38e-06 0;-7.37e-06 0;-7.36e-06 0;-7.35e-06 0;-7.34e-06 0;-7.33e-06 0;-7.32e-06 0;-7.31e-06 0;-7.3e-06 0;-7.29e-06 0;-7.28e-06 0;-7.27e-06 0;-7.26e-06 0;-7.25e-06 0;-7.24e-06 0;-7.23e-06 0;-7.22e-06 0;-7.21e-06 0;-7.2e-06 0;-7.19e-06 0;-7.18e-06 0;-7.17e-06 0;-7.16e-06 0;-7.15e-06 0;-7.14e-06 0;-7.13e-06 0;-7.12e-06 0;-7.11e-06 0;-7.1e-06 0;-7.09e-06 0;-7.08e-06 0;-7.07e-06 0;-7.06e-06 0;-7.05e-06 0;-7.04e-06 0;-7.03e-06 0;-7.02e-06 0;-7.01e-06 0;-7e-06 0;-6.99e-06 0;-6.98e-06 0;-6.97e-06 0;-6.96e-06 0;-6.95e-06 0;-6.94e-06 0;-6.93e-06 0;-6.92e-06 0;-6.91e-06 0;-6.9e-06 0;-6.89e-06 0;-6.88e-06 0;-6.87e-06 0;-6.86e-06 0;-6.85e-06 0;-6.84e-06 0;-6.83e-06 0;-6.82e-06 0;-6.81e-06 0;-6.8e-06 0;-6.79e-06 0;-6.78e-06 0;-6.77e-06 0;-6.76e-06 0;-6.75e-06 0;-6.74e-06 0;-6.73e-06 0;-6.72e-06 0;-6.71e-06 0;-6.7e-06 0;-6.69e-06 0;-6.68e-06 0;-6.67e-06 0;-6.66e-06 0;-6.65e-06 0;-6.64e-06 0;-6.63e-06 0;-6.62e-06 0;-6.61e-06 0;-6.6e-06 0;-6.59e-06 0;-6.58e-06 0;-6.57e-06 0;-6.56e-06 0 ...(+7657 chars)]  x4=[-9.91e-06 0;-9.9e-06 0;-9.89e-06 0;-9.88e-06 0;-9.87e-06 0;-9.86e-06 0;-9.85e-06 0;-9.84e-06 0;-9.83e-06 0;-9.82e-06 0;-9.81e-06 0;-9.8e-06 0;-9.79e-06 0;-9.78e-06 0;-9.77e-06 0;-9.76e-06 0;-9.75e-06 0;-9.74e-06 0;-9.73e-06 0;-9.72e-06 0;-9.71e-06 0;-9.7e-06 0;-9.69e-06 0;-9.68e-06 0;-9.67e-06 0;-9.66e-06 0;-9.65e-06 0;-9.64e-06 0;-9.63e-06 0;-9.62e-06 0;-9.61e-06 0;-9.6e-06 0;-9.59e-06 0;-9.58e-06 0;-9.57e-06 0;-9.56e-06 0;-9.55e-06 0;-9.54e-06 0;-9.53e-06 0;-9.52e-06 0;-9.51e-06 0;-9.5e-06 0;-9.49e-06 0;-9.48e-06 0;-9.47e-06 0;-9.46e-06 0;-9.45e-06 0;-9.44e-06 0;-9.43e-06 0;-9.42e-06 0;-9.41e-06 0;-9.4e-06 0;-9.39e-06 0;-9.38e-06 0;-9.37e-06 0;-9.36e-06 0;-9.35e-06 0;-9.34e-06 0;-9.33e-06 0;-9.32e-06 0;-9.31e-06 0;-9.3e-06 0;-9.29e-06 0;-9.28e-06 0;-9.27e-06 0;-9.26e-06 0;-9.25e-06 0;-9.24e-06 0;-9.23e-06 0;-9.22e-06 0;-9.21e-06 0;-9.2e-06 0;-9.19e-06 0;-9.18e-06 0;-9.17e-06 0;-9.16e-06 0;-9.15e-06 0;-9.14e-06 0;-9.13e-06 0;-9.12e-06 0;-9.11e-06 0;-9.1e-06 0;-9.09e-06 0;-9.08e-06 0;-9.07e-06 0;-9.06e-06 0;-9.05e-06 0;-9.04e-06 0;-9.03e-06 0;-9.02e-06 0;-9.01e-06 0;-9e-06 0;-8.99e-06 0;-8.98e-06 0;-8.97e-06 0;-8.96e-06 0;-8.95e-06 0;-8.94e-06 0;-8.93e-06 0;-8.92e-06 0;-8.91e-06 0;-8.9e-06 0;-8.89e-06 0;-8.88e-06 0;-8.87e-06 0;-8.86e-06 0;-8.85e-06 0;-8.84e-06 0;-8.83e-06 0;-8.82e-06 0;-8.81e-06 0;-8.8e-06 0;-8.79e-06 0;-8.78e-06 0;-8.77e-06 0;-8.76e-06 0;-8.75e-06 0;-8.74e-06 0;-8.73e-06 0;-8.72e-06 0;-8.71e-06 0;-8.7e-06 0;-8.69e-06 0;-8.68e-06 0;-8.67e-06 0;-8.66e-06 0;-8.65e-06 0;-8.64e-06 0;-8.63e-06 0;-8.62e-06 0;-8.61e-06 0;-8.6e-06 0;-8.59e-06 0;-8.58e-06 0;-8.57e-06 0;-8.56e-06 0;-8.55e-06 0;-8.54e-06 0;-8.53e-06 0;-8.52e-06 0;-8.51e-06 0;-8.5e-06 0;-8.49e-06 0;-8.48e-06 0;-8.47e-06 0;-8.46e-06 0;-8.45e-06 0;-8.44e-06 0;-8.43e-06 0;-8.42e-06 0;-8.41e-06 0;-8.4e-06 0;-8.39e-06 0;-8.38e-06 0;-8.37e-06 0;-8.36e-06 0;-8.35e-06 0;-8.34e-06 0;-8.33e-06 0;-8.32e-06 0;-8.31e-06 0;-8.3e-06 0;-8.29e-06 0;-8.28e-06 0;-8.27e-06 0;-8.26e-06 0;-8.25e-06 0;-8.24e-06 0;-8.23e-06 0;-8.22e-06 0;-8.21e-06 0;-8.2e-06 0;-8.19e-06 0;-8.18e-06 0;-8.17e-06 0;-8.16e-06 0;-8.15e-06 0;-8.14e-06 0;-8.13e-06 0;-8.12e-06 0;-8.11e-06 0;-8.1e-06 0;-8.09e-06 0;-8.08e-06 0;-8.07e-06 0;-8.06e-06 0;-8.05e-06 0;-8.04e-06 0;-8.03e-06 0;-8.02e-06 0;-8.01e-06 0;-8e-06 0;-7.99e-06 0;-7.98e-06 0;-7.97e-06 0;-7.96e-06 0;-7.95e-06 0;-7.94e-06 0;-7.93e-06 0;-7.92e-06 0;-7.91e-06 0;-7.9e-06 0;-7.89e-06 0;-7.88e-06 0;-7.87e-06 0;-7.86e-06 0;-7.85e-06 0;-7.84e-06 0;-7.83e-06 0;-7.82e-06 0;-7.81e-06 0;-7.8e-06 0;-7.79e-06 0;-7.78e-06 0;-7.77e-06 0;-7.76e-06 0;-7.75e-06 0;-7.74e-06 0;-7.73e-06 0;-7.72e-06 0;-7.71e-06 0;-7.7e-06 0;-7.69e-06 0;-7.68e-06 0;-7.67e-06 0;-7.66e-06 0;-7.65e-06 0;-7.64e-06 0;-7.63e-06 0;-7.62e-06 0;-7.61e-06 0;-7.6e-06 0;-7.59e-06 0;-7.58e-06 0;-7.57e-06 0;-7.56e-06 0;-7.55e-06 0;-7.54e-06 0;-7.53e-06 0;-7.52e-06 0;-7.51e-06 0;-7.5e-06 0;-7.49e-06 0;-7.48e-06 0;-7.47e-06 0;-7.46e-06 0;-7.45e-06 0;-7.44e-06 0;-7.43e-06 0;-7.42e-06 0;-7.41e-06 0;-7.4e-06 0;-7.39e-06 0;-7.38e-06 0;-7.37e-06 0;-7.36e-06 0;-7.35e-06 0;-7.34e-06 0;-7.33e-06 0;-7.32e-06 0;-7.31e-06 0;-7.3e-06 0;-7.29e-06 0;-7.28e-06 0;-7.27e-06 0;-7.26e-06 0;-7.25e-06 0;-7.24e-06 0;-7.23e-06 0;-7.22e-06 0;-7.21e-06 0;-7.2e-06 0;-7.19e-06 0;-7.18e-06 0;-7.17e-06 0;-7.16e-06 0;-7.15e-06 0;-7.14e-06 0;-7.13e-06 0;-7.12e-06 0;-7.11e-06 0;-7.1e-06 0;-7.09e-06 0;-7.08e-06 0;-7.07e-06 0;-7.06e-06 0;-7.05e-06 0;-7.04e-06 0;-7.03e-06 0;-7.02e-06 0;-7.01e-06 0;-7e-06 0;-6.99e-06 0;-6.98e-06 0;-6.97e-06 0;-6.96e-06 0;-6.95e-06 0;-6.94e-06 0;-6.93e-06 0;-6.92e-06 0;-6.91e-06 0;-6.9e-06 0;-6.89e-06 0;-6.88e-06 0;-6.87e-06 0;-6.86e-06 0;-6.85e-06 0;-6.84e-06 0;-6.83e-06 0;-6.82e-06 0;-6.81e-06 0;-6.8e-06 0;-6.79e-06 0;-6.78e-06 0;-6.77e-06 0;-6.76e-06 0;-6.75e-06 0;-6.74e-06 0;-6.73e-06 0;-6.72e-06 0;-6.71e-06 0;-6.7e-06 0;-6.69e-06 0;-6.68e-06 0;-6.67e-06 0;-6.66e-06 0;-6.65e-06 0;-6.64e-06 0;-6.63e-06 0;-6.62e-06 0;-6.61e-06 0;-6.6e-06 0;-6.59e-06 0;-6.58e-06 0;-6.57e-06 0;-6.56e-06 0 ...(+7657 chars)]  x5=9.90111104876619e-06  V1=[0;0;1.571]  V2=[0;0;1.571]  I1=[0;0;1.571]  I2=[0;0;1.571]  nHarmo=1  Measurements=Phase-to-ground voltages
  Ground : powerlib/Elements/Ground  LConnTagsString=a
  Ground1 : powerlib/Elements/Ground  LConnTagsString=a
  Ground2 : powerlib/Elements/Ground  LConnTagsString=a
  Scope{,1..3} (4 alike) : Scope
  Series RLC Branch : powerlib/Elements/Series RLC Branch  LConnTagsString=__new0  RConnTagsString=__new0  BranchType=R  Resistance=10000  Inductance=1e-3  SetiL0=off  InitialCurrent=0  Capacitance=1e-6  Setx0=off  InitialVoltage=0  Measurements=Branch voltage
  Series RLC Branch1 : powerlib/Elements/Series RLC Branch  LConnTagsString=__new0  RConnTagsString=__new0  BranchType=R  Resistance=1  Inductance=1e-3  SetiL0=off  InitialCurrent=0  Capacitance=1e-6  Setx0=off  InitialVoltage=0  Measurements=Branch voltage
  Series RLC Branch2 : powerlib/Elements/Series RLC Branch  LConnTagsString=__new0  RConnTagsString=__new0  BranchType=R  Resistance=0.001  Inductance=1e-3  SetiL0=off  InitialCurrent=0  Capacitance=1e-6  Setx0=off  InitialVoltage=0  Measurements=Branch voltage
  Step : Step  Time=0.3E-6  Before=28  After=0  SampleTime=1E-08
  Step1 : Step  Time=0.1E-6  Before=-28  After=0  SampleTime=1E-08
  Voltage Measurement : powerlib/Measurements/Voltage Measurement  PhasorSimulation=off  OutputType=Complex  PSBequivalent=0
  Voltage Measurement1 : powerlib/Measurements/Voltage Measurement  PhasorSimulation=off  OutputType=Complex  PSBequivalent=0
  Voltage Measurement2 : powerlib/Measurements/Voltage Measurement  PhasorSimulation=off  OutputType=Complex  PSBequivalent=0
  powergui : powerlib/powergui  Priority=1  SimulationMode=Discrete  SolverType=Tustin/Backward Euler (TBE)  SampleTime=0.01e-6  frequency=60  SPID=off  DisableSnubberDevices=off  DisableRonSwitches=off  DisableVfSwitches=off  SwTol=0  DisplayEquations=off  Interpol=off  ExternalGateDelay=off  methode=off  Ts=100  FunctionMessages=off  echomessages=off  HookPort=off  EnableUseOfTLC=off  x0status=blocks  frequencyindice=0  Pbase=100e6  ErrMax=1e-4  Iterations=50  UnitsV=V  UnitsW=W  buscounter=0  RestoreLinks=warning  ResistiveCurrentMeasurement=off  Frange=[0:2:500]  Ylog=off  Xlog=on  ShowGrid=off  save=off  variable=ZData  structure=0  ZoomFFT=off  StartTime=0.0  cycles=1  DisplayStyle=1  fundamental=60  FreqAxis=off  MaxFrequency=1000  frequencyindicesteady=1  RmsSteady=1  display=off
  wires:
  Voltage Measurement/1 -> Scope/1
  Voltage Measurement1/1 -> Scope1/1
  Step/1 -> Add/1
  Step1/1 -> Add/2
  Add/1 -> Controlled Voltage Source1/1, Scope2/1
  Voltage Measurement2/1 -> Scope3/1
  connections:
  Distributed Parameters Line1/RConn1 -- Series RLC Branch2/LConn1 -- Breaker/LConn1
  Voltage Measurement/LConn2 -- Series RLC Branch2/RConn1 -- Controlled Voltage Source1/LConn1 -- Voltage Measurement1/LConn2 -- Ground/LConn1
  Series RLC Branch/LConn1 -- Distributed Parameters Line2/RConn1 -- Voltage Measurement2/LConn1
  Ground1/LConn1 -- Series RLC Branch/RConn1
  Controlled Voltage Source1/RConn1 -- Series RLC Branch1/LConn1 -- Voltage Measurement1/LConn1
  Ground2/LConn1 -- Voltage Measurement2/LConn2
  Series RLC Branch1/RConn1 -- Voltage Measurement/LConn1 -- Distributed Parameters Line1/LConn1
  Breaker/RConn1 -- Distributed Parameters Line2/LConn1
